simulink model "DCMotor_model_comparison_PID_librarymodel"  (R2021a)
settings: Solver=VariableStepAuto  StartTime=0.0  StopTime=10  MaxStep=0.0001  RelTol=1e-5
PostLoadFcn:
  | % Resize the model window
  | set(0,"Units","pixels")
  | sSize = get(0,"screensize");
  | set_param(gcs,'location',...
  |     [1,sSize(4)*0.01,round(sSize(3)/2),sSize(4)*0.96]);
  | 
  | % Reset the zoom
  | set_param(gcs, 'ZoomFactor','FitSystem')
libraries: PlantLibrary x1
settings Model: Creator=Rocksmithed  LastModifiedBy=Work
settings ExplorerConfigSet: InternalSimMechanicsExplorerSettings="<ExplorerConfiguration><canonicalview>default</canonicalview><AnimationSetting><BasePlaybackSpeed>1.0</BasePlaybackSpeed><PlaybackSpeedFactor>1.0</PlaybackSpeedFactor></AnimationSetting><TilePanel><TileInfo><Tiles Columns=\"1\" Count=\"2\" Rows=\"2\"><Column Weight=\"1\"/><Row Weight=\"0.567\"/><Row Weight=\"0.433\"/><Tile Height=\"1\" Width=\"1\" X=\"0\" Y=\"0\"/><Tile Height=\"1\" Width=\"1\" X=\"0\" Y=\"1\"/></Tiles></TileInfo><SceneInfo><SceneViewer><BGColor><R>0.556862771511077881</R><G>0.556862771511077881</G><B>0.556862771511077881</B></BGColor><Camera><DoPerspective>off</DoPerspective><Position><X>-0.000930544299837629606</X><Y>-0.991947113333839781</Y><Z>-0.000895731694159566396</Z></Position><Center><X>-0.000930544299837629606</X><Y>0.00805288666616021942</Y><Z>-0.000895731694159566396</Z></Center><Up><X>0</X><Y>-0</Y><Z>1</Z></Up><ViewLimDist>1</ViewLimDist><YLim>0.0189692402762493932</YLim><XLim>0.040223097082120067</XLim></Camera></SceneViewer><SceneViewer><BGColor><R>0.556862771511077881</R><G>0.556862771511077881</G><B>0.556862771511077881</B></BGColor><Camera><DoPerspective>off</DoPerspective><Position><X>0.999997946466442578</X><Y>0.00754476683050594576</Y><Z>-0.00157074132845253563</Z></Position><Center><X>-2.05353355742232679e-06</X><Y>0.00754476683050594576</Y><Z>-0.00157074132845253563</Z></Center><Up><X>-0</X><Y>0</Y><Z>1</Z></Up><ViewLimDist>1</ViewLimDist><YLim>0.0170723162486244549</YLim><XLim>0.0475352192034383808</XLim></Camera></SceneViewer></SceneInfo></TilePanel><MechEditorPanel><Cameras/><GfxPanelCameraMap/><VideoCreator><PlaybackSpeedRatio>1.0</PlaybackSpeedRatio><FrameRate>30</FrameRate><VideoFormat>Motion JPEG AVI</VideoFormat><FrameSize>auto</FrameSize></VideoCreator></MechEditorPanel></ExplorerConfiguration>"

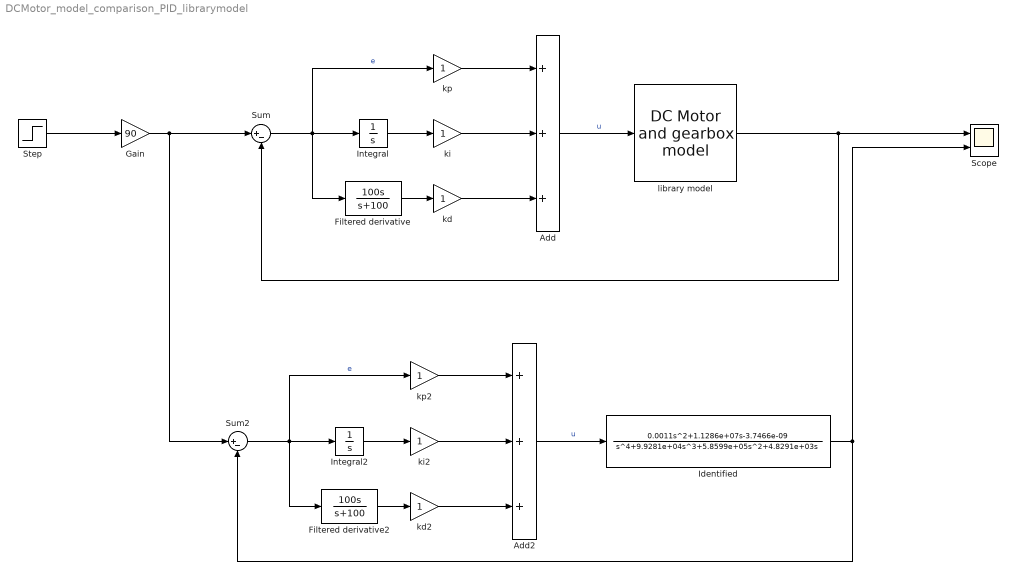
== system DCMotor_model_comparison_PID_librarymodel ==
  Add : Sum  Inputs=+++
  Add2 : Sum  Inputs=+++
  Filtered derivative : TransferFcn  Numerator=[100 0]  Denominator=[1 100]
  Filtered derivative2 : TransferFcn  Numerator=[100 0]  Denominator=[1 100]
  Gain : Gain  Gain=90
  Identified : TransferFcn  Numerator=[0 0 0.0011 1.1286e+07 -3.7466e-09]  Denominator=[1 9.9281e+04 5.8599e+05 4.8291e+03 0]
  Integral : Integrator
  Integral2 : Integrator
  Scope : Scope  NumInputPorts=2
  Step : Step  SampleTime=0
  Sum : Sum  Inputs=|+-
  Sum2 : Sum  Inputs=|+-
  kd : Gain
  kd2 : Gain
  ki : Gain
  ki2 : Gain
  kp : Gain
  kp2 : Gain
  library model : PlantLibrary/DC Motor and gearbox model  C=0.028  K=0.05  L=0.1  R=0.5  saturationOn=off  pmass=0.300  plength=0.015
  wires:
  Add/1 -> library model/1  "u"
  kp/1 -> Add/1
  ki/1 -> Add/2
  kd/1 -> Add/3
  Integral/1 -> ki/1
  Filtered derivative/1 -> kd/1
  Sum/1 -> kp/1, Filtered derivative/1, Integral/1  "e"
  library model/1 -> Sum/2, Scope/1
  Step/1 -> Gain/1
  Gain/1 -> Sum2/1, Sum/1
  Sum2/1 -> kp2/1, Filtered derivative2/1, Integral2/1  "e"
  Integral2/1 -> ki2/1
  ki2/1 -> Add2/2
  kp2/1 -> Add2/1
  Filtered derivative2/1 -> kd2/1
  kd2/1 -> Add2/3
  Add2/1 -> Identified/1  "u"
  Identified/1 -> Scope/2, Sum2/2
